simulink model "outerloop"  (Simulink 7.3)
settings: Solver=ode45  StartTime=0.0  StopTime=300  RelTol=1e-3
values from neighbouring files (symbols this model uses):
  Ts = 0.02    [process_ol.m]    (also in process_ol_data.m)
settings Model: Creator=Administrator  LastModifiedBy=Administrator

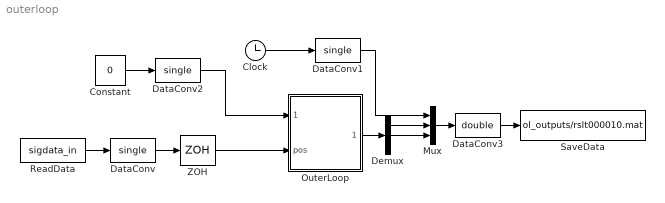
== system outerloop ==
  Clock : Clock
  Constant : Constant  Value=0  OutDataType=fixdt(1, 16)  OutScaling=2^0
  DataConv : DataTypeConversion  OutDataTypeMode=single  OutDataType=single\  OutDataTypeStr=single
  DataConv1 : DataTypeConversion  OutDataTypeMode=single  OutDataType=single\  OutDataTypeStr=single
  DataConv2 : DataTypeConversion  OutDataTypeMode=single  OutDataType=single\  OutDataTypeStr=single
  DataConv3 : DataTypeConversion  OutDataTypeMode=double  OutDataType=single\  OutDataTypeStr=double
  Demux : Demux  Outputs=5
  Mux : Mux  Inputs=3
  OuterLoop : Subsystem
  ReadData : FromWorkspace  VariableName=sigdata_in  SampleTime=0
  SaveData : ToFile  Filename=ol_outputs/rslt000010.mat  MatrixName=sigdata_out
  ZOH : ZeroOrderHold  SampleTime=Ts
  wires:
  ReadData/1 -> DataConv/1
  Constant/1 -> DataConv2/1
  DataConv/1 -> ZOH/1
  OuterLoop/1(ang_ref) -> Demux/1
  Demux/1 -> Mux/2
  Demux/3 -> Mux/3
  Mux/1 -> DataConv3/1
  ZOH/1 -> OuterLoop/2(pos)
  Clock/1 -> DataConv1/1
  DataConv1/1 -> Mux/1
  DataConv2/1 -> OuterLoop/1(pos_ref)
  DataConv3/1 -> SaveData/1

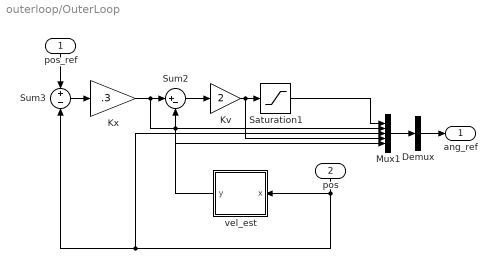
== system outerloop/OuterLoop ==
  pos_ref : Inport  PortDimensions=1  DataType=single  OutDataTypeStr=single
  pos : Inport  Port=2  PortDimensions=1  DataType=single  OutDataTypeStr=single
  Demux : Demux  Outputs=1
  Kv : Gain  Gain=2  ParameterDataTypeMode=single  ParameterDataType=sfix(16)  ParameterScaling=2^0  ParamDataTypeStr=single  OutDataType=sfix(16)  OutScaling=2^0
  Kx : Gain  Gain=.3  ParameterDataTypeMode=single  ParameterDataType=sfix(16)  ParameterScaling=2^0  ParamDataTypeStr=single  OutDataType=sfix(16)  OutScaling=2^0
  Mux1 : Mux  Inputs=5
  Saturation1 : Saturate  UpperLimit=pi/4  LowerLimit=-pi/4  OutDataType=sfix(16)  OutScaling=2^0
  Sum2 : Sum  Inputs=|+-  OutDataType=sfix(16)  OutScaling=2^0
  Sum3 : Sum  Inputs=+|-  OutDataType=sfix(16)  OutScaling=2^0
  vel_est : Subsystem
  ang_ref : Outport  DataType=single  OutDataTypeStr=single
  wires:
  Kx/1 -> Sum2/1, Mux1/2
  Sum2/1 -> Kv/1
  Kv/1 -> Saturation1/1, Mux1/4
  vel_est/1(y) -> Sum2/2, Mux1/5
  Sum3/1 -> Kx/1
  pos_ref/1 -> Sum3/1
  pos/1 -> vel_est/1(x), Sum3/2, Mux1/3
  Mux1/1 -> Demux/1
  Saturation1/1 -> Mux1/1
  Demux/1 -> ang_ref/1

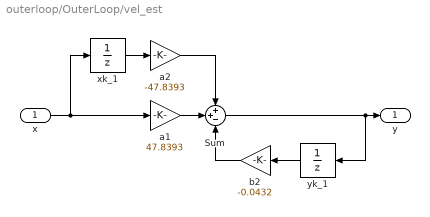
== system outerloop/OuterLoop/vel_est ==
  x : Inport  PortDimensions=1  DataType=single  OutDataType=sfix(16)  OutScaling=2^0  OutDataTypeStr=single
  Sum : Sum  Inputs=++-  OutDataType=sfix(16)  OutScaling=2^0
  a1 : Gain  Gain=47.8393  ParameterDataTypeMode=single  ParameterDataType=sfix(16)  ParameterScaling=2^0  ParamDataTypeStr=single  OutDataType=sfix(16)  OutScaling=2^0
  a2 : Gain  Gain=-47.8393  ParameterDataTypeMode=single  ParameterDataType=sfix(16)  ParameterScaling=2^0  ParamDataTypeStr=single  OutDataType=sfix(16)  OutScaling=2^0
  b2 : Gain  Gain=-0.0432  ParameterDataTypeMode=single  ParameterDataType=sfix(16)  ParameterScaling=2^0  ParamDataTypeStr=single  OutDataType=sfix(16)  OutScaling=2^0
  xk_1 : UnitDelay  SampleTime=Ts
  yk_1 : UnitDelay  SampleTime=Ts
  y : Outport  OutDataType=sfix(16)  OutScaling=2^0
  wires:
  x/1 -> a1/1, xk_1/1
  xk_1/1 -> a2/1
  a2/1 -> Sum/1
  a1/1 -> Sum/2
  Sum/1 -> yk_1/1, y/1
  yk_1/1 -> b2/1
  b2/1 -> Sum/3
